simulink model "Model"  (R2023b)
settings: Solver=FixedStepAuto  StartTime=0.0  StopTime=10  FixedStep=0.002  RelTol=1e-3
undefined symbols (not defined in the file or in its folder): K, X, Y, Z
libraries: sm_lib x47, nesl_utility x15, simulink x2, slpidlib x2
(part 1 of 4)
settings Model: Creator=Mas  LastModifiedBy=Mas

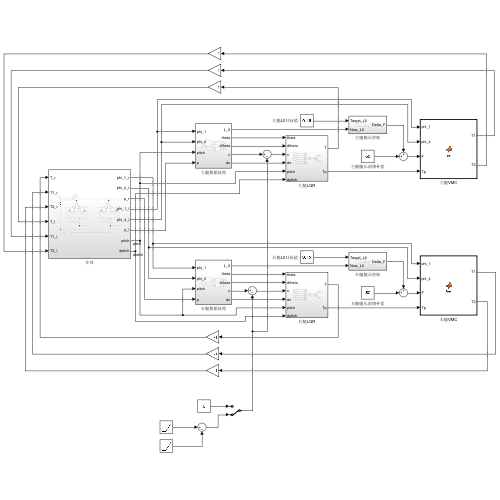
[thumbnail: Simulink's stored preview of the top-level diagram]
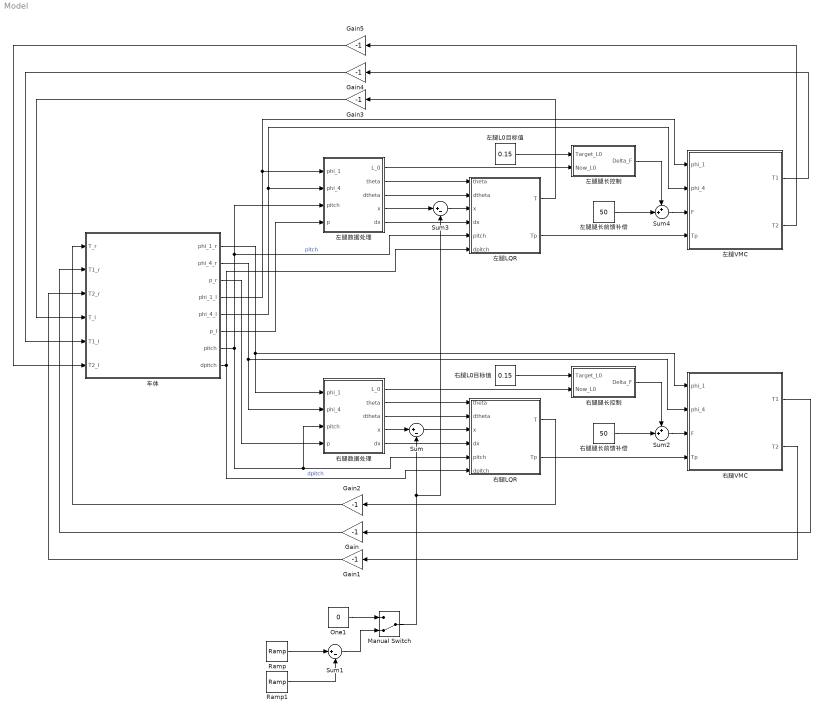
== system Model ==
  Gain{,1..5} (6 alike) : Gain  Gain=-1
  Manual Switch : ManualSwitch  CurrentSetting=0
  One1 : Constant  Value=0  OutDataTypeStr=Inherit: Inherit via back propagation
  Ramp : simulink/Sources/Ramp  slope=2  start=1  InitialOutput=0
  Ramp1 : simulink/Sources/Ramp  slope=2  start=2  InitialOutput=0
  Sum : Sum  Inputs=|+-
  Sum1 : Sum  Inputs=|+-
  Sum2 : Sum  Inputs=++|
  Sum3 : Sum  Inputs=|+-
  Sum4 : Sum  Inputs=++|
  右腿L0目标值 : Constant  Value=0.15  OutDataTypeStr=Inherit: Inherit via back propagation
  右腿LQR : Subsystem
  右腿VMC : MATLAB Function  TreatAsAtomicUnit=on
  右腿数据处理 : Subsystem
  右腿腿长前馈补偿 : Constant  Value=50  OutDataTypeStr=Inherit: Inherit via back propagation
  右腿腿长控制 : Subsystem
  左腿L0目标值 : Constant  Value=0.15  OutDataTypeStr=Inherit: Inherit via back propagation
  左腿LQR : Subsystem
  左腿VMC : MATLAB Function  TreatAsAtomicUnit=on
  左腿数据处理 : Subsystem
  左腿腿长前馈补偿 : Constant  Value=50  OutDataTypeStr=Inherit: Inherit via back propagation
  左腿腿长控制 : Subsystem
  车体 : Subsystem
  wires:
  右腿VMC/2(T2) -> Gain1/1
  右腿VMC/1(T1) -> Gain/1
  右腿LQR/1(T) -> Gain2/1
  右腿LQR/2(Tp) -> 右腿VMC/4(Tp)
  Sum/1 -> 右腿LQR/3(x)
  右腿腿长前馈补偿/1 -> Sum2/2
  右腿腿长控制/1(Delta_F) -> Sum2/1
  右腿L0目标值/1 -> 右腿腿长控制/1(Target_L0)
  Sum2/1 -> 右腿VMC/3(F)
  One1/1 -> Manual Switch/1
  Manual Switch/1 -> Sum3/2, Sum/2
  Ramp/1 -> Sum1/1
  Ramp1/1 -> Sum1/2
  Sum1/1 -> Manual Switch/2
  右腿数据处理/1(L_0) -> 右腿腿长控制/2(Now_L0)
  右腿数据处理/2(theta) -> 右腿LQR/1(theta)
  右腿数据处理/3(dtheta) -> 右腿LQR/2(dtheta)
  右腿数据处理/5(dx) -> 右腿LQR/4(dx)
  右腿数据处理/4(x) -> Sum/1
  Gain2/1 -> 车体/1(T_r)
  Gain/1 -> 车体/2(T1_r)
  Gain1/1 -> 车体/3(T2_r)
  车体/7(pitch) -> 右腿数据处理/3(pitch), 右腿LQR/5(pitch), 左腿数据处理/3(pitch), 左腿LQR/5(pitch)  "pitch"
  车体/8(dpitch) -> 左腿LQR/6(dpitch), 右腿LQR/6(dpitch)  "dpitch"
  车体/1(phi_1_r) -> 右腿VMC/1(phi_1), 右腿数据处理/1(phi_1)
  车体/2(phi_4_r) -> 右腿VMC/2(phi_4), 右腿数据处理/2(phi_4)
  车体/3(p_r) -> 右腿数据处理/4(p)
  车体/4(phi_1_l) -> 左腿VMC/1(phi_1), 左腿数据处理/1(phi_1)
  车体/5(phi_4_l) -> 左腿VMC/2(phi_4), 左腿数据处理/2(phi_4)
  车体/6(p_l) -> 左腿数据处理/4(p)
  左腿数据处理/2(theta) -> 左腿LQR/1(theta)
  左腿数据处理/3(dtheta) -> 左腿LQR/2(dtheta)
  左腿数据处理/5(dx) -> 左腿LQR/4(dx)
  Sum3/1 -> 左腿LQR/3(x)
  左腿数据处理/4(x) -> Sum3/1
  左腿数据处理/1(L_0) -> 左腿腿长控制/2(Now_L0)
  左腿L0目标值/1 -> 左腿腿长控制/1(Target_L0)
  左腿LQR/2(Tp) -> 左腿VMC/4(Tp)
  Sum4/1 -> 左腿VMC/3(F)
  左腿腿长前馈补偿/1 -> Sum4/2
  左腿腿长控制/1(Delta_F) -> Sum4/1
  左腿LQR/1(T) -> Gain3/1
  左腿VMC/1(T1) -> Gain4/1
  左腿VMC/2(T2) -> Gain5/1
  Gain3/1 -> 车体/4(T_l)
  Gain4/1 -> 车体/5(T1_l)
  Gain5/1 -> 车体/6(T2_l)

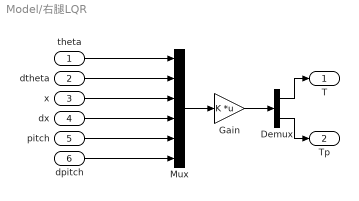
== system Model/右腿LQR ==
  theta : Inport
  dtheta : Inport  Port=2
  x : Inport  Port=3
  dx : Inport  Port=4
  pitch : Inport  Port=5
  dpitch : Inport  Port=6
  Demux : Demux  Outputs=2
  Gain : Gain  Gain=K  Multiplication=Matrix(K*u)
  Mux : Mux  Inputs=6
  T : Outport
  Tp : Outport  Port=2
  wires:
  dtheta/1 -> Mux/2
  theta/1 -> Mux/1
  x/1 -> Mux/3
  dx/1 -> Mux/4
  pitch/1 -> Mux/5
  dpitch/1 -> Mux/6
  Mux/1 -> Gain/1
  Gain/1 -> Demux/1
  Demux/2 -> Tp/1
  Demux/1 -> T/1

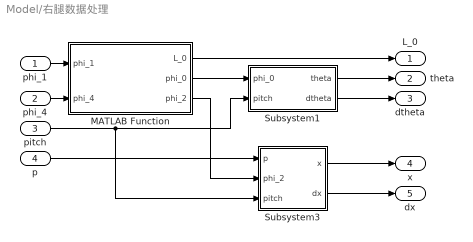
== system Model/右腿数据处理 ==
  phi_1 : Inport
  phi_4 : Inport  Port=2
  pitch : Inport  Port=3
  p : Inport  Port=4
  MATLAB Function : MATLAB Function  TreatAsAtomicUnit=on
  Subsystem1 : Subsystem
  Subsystem3 : Subsystem
  L_0 : Outport
  theta : Outport  Port=2
  dtheta : Outport  Port=3
  x : Outport  Port=4
  dx : Outport  Port=5
  wires:
  Subsystem3/2(dx) -> dx/1
  MATLAB Function/2(phi_0) -> Subsystem1/1(phi_0)
  Subsystem3/1(x) -> x/1
  phi_1/1 -> MATLAB Function/1(phi_1)
  MATLAB Function/3(phi_2) -> Subsystem3/2(phi_2)
  Subsystem1/2(dtheta) -> dtheta/1
  MATLAB Function/1(L_0) -> L_0/1
  Subsystem1/1(theta) -> theta/1
  p/1 -> Subsystem3/1(p)
  phi_4/1 -> MATLAB Function/2(phi_4)
  pitch/1 -> Subsystem3/3(pitch), Subsystem1/2(pitch)

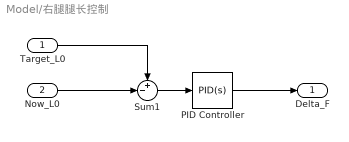
== system Model/右腿腿长控制 ==
  Target_L0 : Inport
  Now_L0 : Inport  Port=2
  PID Controller : slpidlib/PID Controller  Controller=PID  Form=Parallel  TimeDomain=Continuous-time  UseExternalTs=off  SampleTime=-1  IntegratorMethod=Forward Euler  FilterMethod=Forward Euler  ControllerParametersSource=internal  P=1000  I=1000  UseKiTs=off  D=150  N=100  UseFilter=on  TunerSelectOption=Transfer Function Based (PID Tuner App)  InitialConditionSource=internal  InitialConditionForIntegrator=0  InitialConditionForFilter=0  DifferentiatorICPrevScaledInput=0  ExternalReset=none  TrackingMode=off  Kt=1  LimitOutput=off  SatLimitsSource=internal  UpperSaturationLimit=inf  LowerSaturationLimit=-inf  LinearizeAsGain=on  AntiWindupMode=none  Kb=1  LimitIntegrator=off  UpperIntegratorSaturationLimit=inf  LowerIntegratorSaturationLimit=-inf  POutMin=[]  POutMax=[]  IOutMin=[]  IOutMax=[]  DOutMin=[]  DOutMax=[]  NOutMin=[]  NOutMax=[]  SumOutMin=[]  SumOutMax=[]  SaturationOutMin=[]  SaturationOutMax=[]  PParamMin=[]  PParamMax=[]  IParamMin=[]  IParamMax=[]  DParamMin=[]  DParamMax=[]  NParamMin=[]  NParamMax=[]  KbParamMin=[]  KbParamMax=[]  KtParamMin=[]  KtParamMax=[]  KbOutMin=[]  KbOutMax=[]  KtOutMin=[]  KtOutMax=[]  IntegratorOutMin=[]  IntegratorOutMax=[]  FilterOutMin=[]  FilterOutMax=[]  SumI1OutMin=[]  SumI1OutMax=[]  SumI2OutMin=[]  SumI2OutMax=[]  SumI3OutMin=[]  SumI3OutMax=[]  SumI4OutMin=[]  SumI4OutMax=[]  SumDOutMin=[]  SumDOutMax=[]  DifferentiatorOutMin=[]  DifferentiatorOutMax=[]  FilterDiffOutCoefMin=[]  FilterDiffOutCoefMax=[]  ReciprocalOutMin=[]  ReciprocalOutMax=[]  SumDenOutMin=[]  SumDenOutMax=[]  SumNumOutMin=[]  SumNumOutMax=[]  DivideOutMin=[]  DivideOutMax=[]  UdiffTsProdOutMin=[]  UdiffTsProdOutMax=[]  NTsProdOutMin=[]  NTsProdOutMax=[]  UintegralTsProdOutMin=[]  UintegralTsProdOutMax=[]  UngainTsProdOutMin=[]  UngainTsProdOutMax=[]  ClampingZeroOutDataTypeStr=Inherit: Inherit via back propagation  ClampingZeroOutMin=[]  ClampingZeroOutMax=[]  FilterDenConstantOutDataTypeStr=Inherit: Inherit via back propagation  FilterDenConstantOutMin=[]  FilterDenConstantOutMax=[]  PCopyOutDataTypeStr=Inherit: Inherit via back propagation  PCopyOutMin=[]  PCopyOutMax=[]  NCopyOutDataTypeStr=Inherit: Inherit via back propagation  NCopyOutMin=[]  NCopyOutMax=[]  IntegratorContinuousStateAttributes=''  IntegratorStateMustResolveToSignalObject=off  IntegratorRTWStateStorageClass=Auto  FilterContinuousStateAttributes=''  FilterStateMustResolveToSignalObject=off  FilterRTWStateStorageClass=Auto  ParallelPVariant=InternalParameters  IdealPVariant=Disabled  IVariant=InternalParameters  DVariant=InternalParameters  IntegratorVariant=Continuous  SatVariant=Disabled  AWVariant=Passthrough  PCopyVariant=Disabled  TRVariant=Disabled  FdbkBlocksVariant=Forward  IdealPFdbkVariant=Disabled  SatFdbkVariant=Disabled  DerivativeFilterVariant=ContFilter  NVariant=InternalParameters  NCopyVariant=Disabled  FilterICVariant=InternalICsFilter  IntegratorICVariant=InternalICs  ExternalResetVariant=Disabled  TRSumVariant=Passthrough  SumFdbkVariant=Disabled  SumVariant=Sum_PID  TsampFilterVariant=InternalTs  TsampNgainVariant=Passthrough  TsampIntegralVariant=Disabled_SignalSpec  ExternalSaturationOutDataTypeStr=Inherit: Same as second input
  Sum1 : Sum  Inputs=+-|
  Delta_F : Outport
  wires:
  Now_L0/1 -> Sum1/2
  Sum1/1 -> PID Controller/1
  Target_L0/1 -> Sum1/1
  PID Controller/1 -> Delta_F/1

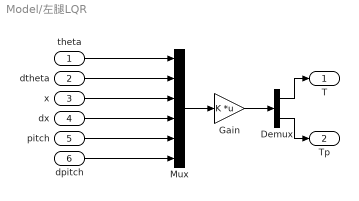
== system Model/左腿LQR ==
  theta : Inport
  dtheta : Inport  Port=2
  x : Inport  Port=3
  dx : Inport  Port=4
  pitch : Inport  Port=5
  dpitch : Inport  Port=6
  Demux : Demux  Outputs=2
  Gain : Gain  Gain=K  Multiplication=Matrix(K*u)
  Mux : Mux  Inputs=6
  T : Outport
  Tp : Outport  Port=2
  wires:
  dtheta/1 -> Mux/2
  theta/1 -> Mux/1
  x/1 -> Mux/3
  dx/1 -> Mux/4
  pitch/1 -> Mux/5
  dpitch/1 -> Mux/6
  Mux/1 -> Gain/1
  Gain/1 -> Demux/1
  Demux/2 -> Tp/1
  Demux/1 -> T/1

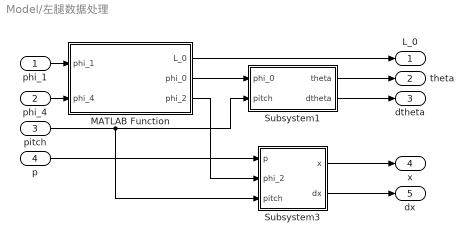
== system Model/左腿数据处理 ==
  phi_1 : Inport
  phi_4 : Inport  Port=2
  pitch : Inport  Port=3
  p : Inport  Port=4
  MATLAB Function : MATLAB Function  TreatAsAtomicUnit=on
  Subsystem1 : Subsystem
  Subsystem3 : Subsystem
  L_0 : Outport
  theta : Outport  Port=2
  dtheta : Outport  Port=3
  x : Outport  Port=4
  dx : Outport  Port=5
  wires:
  Subsystem3/2(dx) -> dx/1
  MATLAB Function/2(phi_0) -> Subsystem1/1(phi_0)
  Subsystem3/1(x) -> x/1
  phi_1/1 -> MATLAB Function/1(phi_1)
  MATLAB Function/3(phi_2) -> Subsystem3/2(phi_2)
  Subsystem1/2(dtheta) -> dtheta/1
  MATLAB Function/1(L_0) -> L_0/1
  Subsystem1/1(theta) -> theta/1
  p/1 -> Subsystem3/1(p)
  phi_4/1 -> MATLAB Function/2(phi_4)
  pitch/1 -> Subsystem3/3(pitch), Subsystem1/2(pitch)

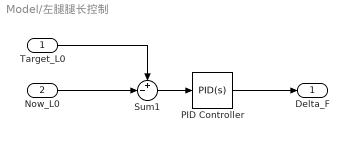
== system Model/左腿腿长控制 ==
  Target_L0 : Inport
  Now_L0 : Inport  Port=2
  PID Controller : slpidlib/PID Controller  Controller=PID  Form=Parallel  TimeDomain=Continuous-time  UseExternalTs=off  SampleTime=-1  IntegratorMethod=Forward Euler  FilterMethod=Forward Euler  ControllerParametersSource=internal  P=1000  I=1000  UseKiTs=off  D=150  N=100  UseFilter=on  TunerSelectOption=Transfer Function Based (PID Tuner App)  InitialConditionSource=internal  InitialConditionForIntegrator=0  InitialConditionForFilter=0  DifferentiatorICPrevScaledInput=0  ExternalReset=none  TrackingMode=off  Kt=1  LimitOutput=off  SatLimitsSource=internal  UpperSaturationLimit=inf  LowerSaturationLimit=-inf  LinearizeAsGain=on  AntiWindupMode=none  Kb=1  LimitIntegrator=off  UpperIntegratorSaturationLimit=inf  LowerIntegratorSaturationLimit=-inf  POutMin=[]  POutMax=[]  IOutMin=[]  IOutMax=[]  DOutMin=[]  DOutMax=[]  NOutMin=[]  NOutMax=[]  SumOutMin=[]  SumOutMax=[]  SaturationOutMin=[]  SaturationOutMax=[]  PParamMin=[]  PParamMax=[]  IParamMin=[]  IParamMax=[]  DParamMin=[]  DParamMax=[]  NParamMin=[]  NParamMax=[]  KbParamMin=[]  KbParamMax=[]  KtParamMin=[]  KtParamMax=[]  KbOutMin=[]  KbOutMax=[]  KtOutMin=[]  KtOutMax=[]  IntegratorOutMin=[]  IntegratorOutMax=[]  FilterOutMin=[]  FilterOutMax=[]  SumI1OutMin=[]  SumI1OutMax=[]  SumI2OutMin=[]  SumI2OutMax=[]  SumI3OutMin=[]  SumI3OutMax=[]  SumI4OutMin=[]  SumI4OutMax=[]  SumDOutMin=[]  SumDOutMax=[]  DifferentiatorOutMin=[]  DifferentiatorOutMax=[]  FilterDiffOutCoefMin=[]  FilterDiffOutCoefMax=[]  ReciprocalOutMin=[]  ReciprocalOutMax=[]  SumDenOutMin=[]  SumDenOutMax=[]  SumNumOutMin=[]  SumNumOutMax=[]  DivideOutMin=[]  DivideOutMax=[]  UdiffTsProdOutMin=[]  UdiffTsProdOutMax=[]  NTsProdOutMin=[]  NTsProdOutMax=[]  UintegralTsProdOutMin=[]  UintegralTsProdOutMax=[]  UngainTsProdOutMin=[]  UngainTsProdOutMax=[]  ClampingZeroOutDataTypeStr=Inherit: Inherit via back propagation  ClampingZeroOutMin=[]  ClampingZeroOutMax=[]  FilterDenConstantOutDataTypeStr=Inherit: Inherit via back propagation  FilterDenConstantOutMin=[]  FilterDenConstantOutMax=[]  PCopyOutDataTypeStr=Inherit: Inherit via back propagation  PCopyOutMin=[]  PCopyOutMax=[]  NCopyOutDataTypeStr=Inherit: Inherit via back propagation  NCopyOutMin=[]  NCopyOutMax=[]  IntegratorContinuousStateAttributes=''  IntegratorStateMustResolveToSignalObject=off  IntegratorRTWStateStorageClass=Auto  FilterContinuousStateAttributes=''  FilterStateMustResolveToSignalObject=off  FilterRTWStateStorageClass=Auto  ParallelPVariant=InternalParameters  IdealPVariant=Disabled  IVariant=InternalParameters  DVariant=InternalParameters  IntegratorVariant=Continuous  SatVariant=Disabled  AWVariant=Passthrough  PCopyVariant=Disabled  TRVariant=Disabled  FdbkBlocksVariant=Forward  IdealPFdbkVariant=Disabled  SatFdbkVariant=Disabled  DerivativeFilterVariant=ContFilter  NVariant=InternalParameters  NCopyVariant=Disabled  FilterICVariant=InternalICsFilter  IntegratorICVariant=InternalICs  ExternalResetVariant=Disabled  TRSumVariant=Passthrough  SumFdbkVariant=Disabled  SumVariant=Sum_PID  TsampFilterVariant=InternalTs  TsampNgainVariant=Passthrough  TsampIntegralVariant=Disabled_SignalSpec  ExternalSaturationOutDataTypeStr=Inherit: Same as second input
  Sum1 : Sum  Inputs=+-|
  Delta_F : Outport
  wires:
  Now_L0/1 -> Sum1/2
  Sum1/1 -> PID Controller/1
  Target_L0/1 -> Sum1/1
  PID Controller/1 -> Delta_F/1
